simulink library "VIS_LIB_backup20190220"  (Simulink 8.6)
settings: Solver=ode45  StartTime=0.0  StopTime=10.0  RelTol=1e-3
undefined symbols (not defined in the file): AC, SIXOSEM_F_WD_AC_MASTER, VIS_LIB, WD2
libraries: cdsEpicsOut x104, cdsTP x55, cdsFilt x52, cdsFiltCtrl x23, cdsRms x23, cdsEpicsIn x16, STATE_BIO_MASTER x5, FOUROSEM_WD_AC_MASTER x4, cdsFunctionCall x2, TYPEB_MASTER x1, cdsEpicsBinIn x1, CRYP_TM_MASTER x1
(part 1 of 9)
settings Model: Creator=keiko  LastModifiedBy=controls

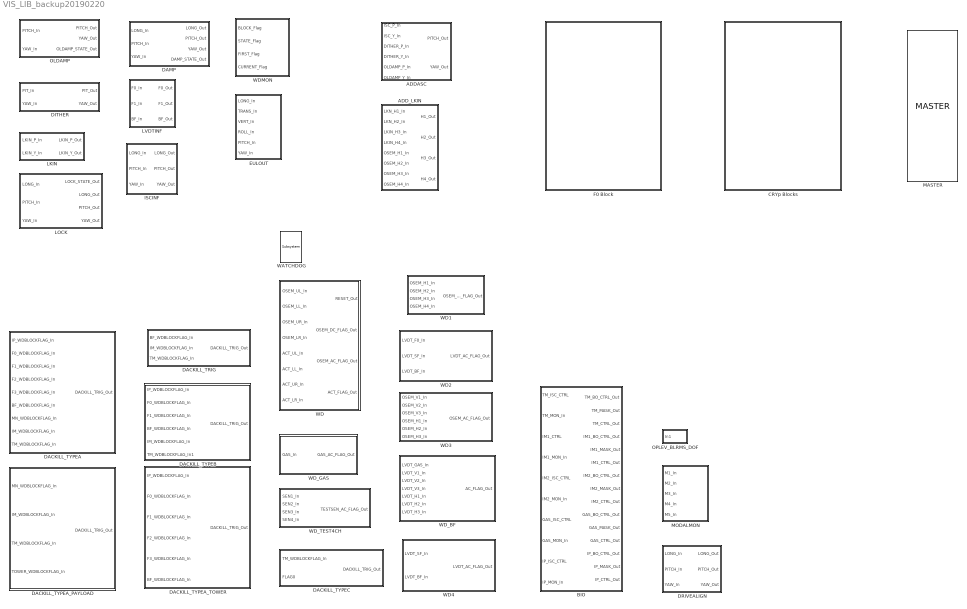
== system VIS_LIB_backup20190220 ==
  ADDASC : Subsystem
  ADD_LKIN : Subsystem
  BIO : Subsystem
  CRYp Blocks : Subsystem
  DACKILL_TRIG : Subsystem
  DACKILL_TYPEA : Subsystem
  DACKILL_TYPEA_PAYLOAD : Subsystem
  DACKILL_TYPEA_TOWER : Subsystem
  DACKILL_TYPEB : Subsystem
  "DACKILL_TYPEC " : Subsystem
  DAMP : Subsystem
  DITHER : Subsystem
  DRIVEALIGN : Subsystem
  EULOUT : Subsystem
  F0 Block : Subsystem
  ISCINF : Subsystem
  LKIN : Subsystem
  LOCK : Subsystem
  LVDTINF : Subsystem
  MASTER : CRYP_TM_MASTER/CRYP_TM_MASTER/MASTER
  MODALMON : Subsystem
  OLDAMP : Subsystem
  OPLEV_BLRMS_DOF : Subsystem
  WATCHDOG : cdsFunctionCall/Subsystem  Tag=cdsFunctionCall  Description=inline OSEMWATCHDOG $SUS_SRC/WATCHDOG.c
      settings: AttributesFormatString=%<Tag>\n%<Description>
  WD : Subsystem
  WD1 : Subsystem
  WD2 : Subsystem
  WD3 : Subsystem
  WD4 : Subsystem  AncestorBlock=VIS_LIB/WD2
  WDMON : Subsystem
  WD_BF : Subsystem
  WD_GAS : Subsystem
  WD_TEST4CH : Subsystem

== system VIS_LIB_backup20190220/ADDASC ==
  ISC_P_In : Inport
  ISC_Y_In : Inport  Port=2
  DITHER_P_In : Inport  Port=3
  DITHER_Y_In : Inport  Port=4
  OLDAMP_P_In : Inport  Port=5
  OLDAMP_Y_In : Inport  Port=6
  Sum3 : Sum  Inputs=+++
  Sum4 : Sum  Inputs=+++
  PITCH_Out : Outport
  YAW_Out : Outport  Port=2
  wires:
  OLDAMP_Y_In/1 -> Sum3/3
  DITHER_Y_In/1 -> Sum3/2
  DITHER_P_In/1 -> Sum4/2
  OLDAMP_P_In/1 -> Sum4/3
  Sum4/1 -> PITCH_Out/1
  ISC_Y_In/1 -> Sum3/1
  ISC_P_In/1 -> Sum4/1
  Sum3/1 -> YAW_Out/1

== system VIS_LIB_backup20190220/ADD_LKIN ==
  LKN_H1_In : Inport
  LKN_H2_In : Inport  Port=2
  LKIN_H3_In : Inport  Port=3
  LKIN_H4_In : Inport  Port=4
  OSEM_H1_In : Inport  Port=5
  OSEM_H2_In : Inport  Port=6
  OSEM_H3_In : Inport  Port=7
  OSEM_H4_In : Inport  Port=8
  Sum{,1,3..4} (4 alike) : Sum
  H1_Out : Outport
  H2_Out : Outport  Port=2
  H3_Out : Outport  Port=3
  H4_Out : Outport  Port=4
  wires:
  LKIN_H4_In/1 -> Sum1/1
  LKIN_H3_In/1 -> Sum3/1
  LKN_H2_In/1 -> Sum4/1
  Sum/1 -> H1_Out/1
  LKN_H1_In/1 -> Sum/1
  OSEM_H1_In/1 -> Sum/2
  Sum3/1 -> H3_Out/1
  Sum4/1 -> H2_Out/1
  OSEM_H3_In/1 -> Sum3/2
  OSEM_H2_In/1 -> Sum4/2
  Sum1/1 -> H4_Out/1
  OSEM_H4_In/1 -> Sum1/2

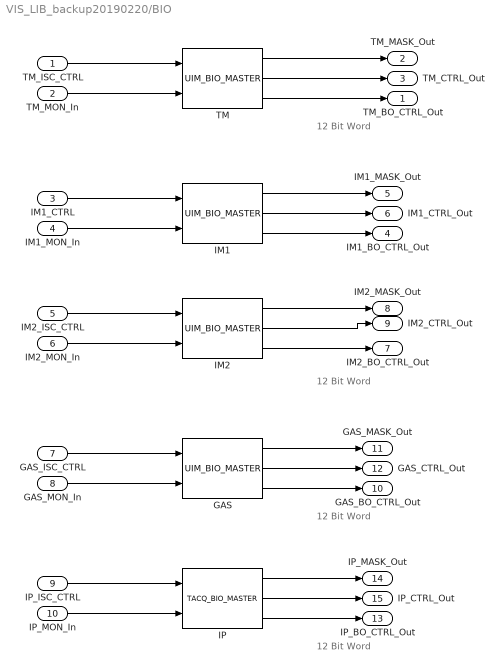
== system VIS_LIB_backup20190220/BIO ==
  note: 12 Bit Word
  note: 12 Bit Word
  note: 12 Bit Word
  note: 12 Bit Word
  TM_ISC_CTRL : Inport
  TM_MON_In : Inport  Port=2
  IM1_CTRL : Inport  Port=3
  IM1_MON_In : Inport  Port=4
  IM2_ISC_CTRL : Inport  Port=5
  IM2_MON_In : Inport  Port=6
  GAS_ISC_CTRL : Inport  Port=7
  GAS_MON_In : Inport  Port=8
  IP_ISC_CTRL : Inport  Port=9
  IP_MON_In : Inport  Port=10
  GAS : STATE_BIO_MASTER/UIM_BIO_MASTER
  IM1 : STATE_BIO_MASTER/UIM_BIO_MASTER
  IM2 : STATE_BIO_MASTER/UIM_BIO_MASTER
  IP : STATE_BIO_MASTER/TACQ_BIO_MASTER
  TM : STATE_BIO_MASTER/UIM_BIO_MASTER
  TM_BO_CTRL_Out : Outport
  TM_MASK_Out : Outport  Port=2
  TM_CTRL_Out : Outport  Port=3
  IM1_BO_CTRL_Out : Outport  Port=4
  IM1_MASK_Out : Outport  Port=5
  IM1_CTRL_Out : Outport  Port=6
  IM2_BO_CTRL_Out : Outport  Port=7
  IM2_MASK_Out : Outport  Port=8
  IM2_CTRL_Out : Outport  Port=9
  GAS_BO_CTRL_Out : Outport  Port=10
  GAS_MASK_Out : Outport  Port=11
  GAS_CTRL_Out : Outport  Port=12
  IP_BO_CTRL_Out : Outport  Port=13
  IP_MASK_Out : Outport  Port=14
  IP_CTRL_Out : Outport  Port=15
  wires:
  IP/3 -> IP_BO_CTRL_Out/1
  IP/2 -> IP_CTRL_Out/1
  IP/1 -> IP_MASK_Out/1
  GAS/3 -> GAS_BO_CTRL_Out/1
  GAS/2 -> GAS_CTRL_Out/1
  GAS/1 -> GAS_MASK_Out/1
  IM2/3 -> IM2_BO_CTRL_Out/1
  IM2/2 -> IM2_CTRL_Out/1
  IM2/1 -> IM2_MASK_Out/1
  IM1/3 -> IM1_BO_CTRL_Out/1
  IM1/2 -> IM1_CTRL_Out/1
  IM1/1 -> IM1_MASK_Out/1
  TM/3 -> TM_BO_CTRL_Out/1
  TM/2 -> TM_CTRL_Out/1
  TM/1 -> TM_MASK_Out/1
  IP_ISC_CTRL/1 -> IP/1
  IP_MON_In/1 -> IP/2
  GAS_ISC_CTRL/1 -> GAS/1
  GAS_MON_In/1 -> GAS/2
  IM2_ISC_CTRL/1 -> IM2/1
  IM2_MON_In/1 -> IM2/2
  IM1_MON_In/1 -> IM1/2
  IM1_CTRL/1 -> IM1/1
  TM_ISC_CTRL/1 -> TM/1
  TM_MON_In/1 -> TM/2

== system VIS_LIB_backup20190220/CRYp Blocks ==
  COILOUTF : Subsystem
  MASTER : Subsystem
  PSWD : Subsystem

== system VIS_LIB_backup20190220/DACKILL_TRIG ==
  note: WDBLOCKFLAG is zero (0) if OK,
      | non-zero if BAD
  note: AND is zero  (0) if all stages are OK
      | non-zero if BAD
  BF_WDBLOCKFLAG_In : Inport
  IM_WDBLOCKFLAG_In : Inport  Port=2
  TM_WDBLOCKFLAG_In : Inport  Port=3
  LogicalOperator1 : Logic  Operator=OR  Inputs=3  AllPortsSameDT=off  OutDataTypeStr=boolean
  STATE : cdsEpicsOut/Subsystem  Tag=cdsEpicsOutput  Description=|
      | Purpose:                                          
      | Output a FE signal to an EPICS channel.           
      |                                                   
      | Operation:                                        
      | Takes input value and passes it to EPICS record.  
      |                                                   
      | Usage:                                            
      | Name the part with the desired EPICS rrecord name.
      settings: AttributesFormatString=%<Tag>
  DACKILL_TRIG_Out : Outport
  wires:
  STATE/1 -> DACKILL_TRIG_Out/1
  BF_WDBLOCKFLAG_In/1 -> LogicalOperator1/1
  IM_WDBLOCKFLAG_In/1 -> LogicalOperator1/2
  TM_WDBLOCKFLAG_In/1 -> LogicalOperator1/3
  LogicalOperator1/1 -> STATE/1

== system VIS_LIB_backup20190220/DACKILL_TYPEA ==
  note: WDBLOCKFLAG is zero (0) if OK,
      | non-zero if BAD
  note: AND is zero  (0) if all stages are OK
      | non-zero if BAD
  IP_WDBLOCKFLAG_In : Inport
  F0_WDBLOCKFLAG_In : Inport  Port=2
  F1_WDBLOCKFLAG_In : Inport  Port=3
  F2_WDBLOCKFLAG_In : Inport  Port=4
  F3_WDBLOCKFLAG_In : Inport  Port=5
  BF_WDBLOCKFLAG_In : Inport  Port=6
  MN_WDBLOCKFLAG_In : Inport  Port=7
  IM_WDBLOCKFLAG_In : Inport  Port=8
  TM_WDBLOCKFLAG_In : Inport  Port=9
  LogicalOperator1 : Logic  Operator=OR  Inputs=9  AllPortsSameDT=off  OutDataTypeStr=boolean
  STATE : cdsEpicsOut/Subsystem  Tag=cdsEpicsOutput  Description=|
      | Purpose:                                          
      | Output a FE signal to an EPICS channel.           
      |                                                   
      | Operation:                                        
      | Takes input value and passes it to EPICS record.  
      |                                                   
      | Usage:                                            
      | Name the part with the desired EPICS rrecord name.
      settings: AttributesFormatString=%<Tag>
  DACKILL_TRIG_Out : Outport
  wires:
  STATE/1 -> DACKILL_TRIG_Out/1
  IP_WDBLOCKFLAG_In/1 -> LogicalOperator1/1
  F0_WDBLOCKFLAG_In/1 -> LogicalOperator1/2
  F1_WDBLOCKFLAG_In/1 -> LogicalOperator1/3
  LogicalOperator1/1 -> STATE/1
  IM_WDBLOCKFLAG_In/1 -> LogicalOperator1/8
  BF_WDBLOCKFLAG_In/1 -> LogicalOperator1/6
  TM_WDBLOCKFLAG_In/1 -> LogicalOperator1/9
  MN_WDBLOCKFLAG_In/1 -> LogicalOperator1/7
  F3_WDBLOCKFLAG_In/1 -> LogicalOperator1/5
  F2_WDBLOCKFLAG_In/1 -> LogicalOperator1/4

== system VIS_LIB_backup20190220/DACKILL_TYPEA_PAYLOAD ==
  note: WDBLOCKFLAG is zero (0) if OK,
      | non-zero if BAD
  note: AND is zero  (0) if all stages are OK
      | non-zero if BAD
  MN_WDBLOCKFLAG_In : Inport
  IM_WDBLOCKFLAG_In : Inport  Port=2
  TM_WDBLOCKFLAG_In : Inport  Port=3
  TOWER_WDBLOCKFLAG_In : Inport  Port=4
  LogicalOperator1 : Logic  Operator=OR  Inputs=3  AllPortsSameDT=off  OutDataTypeStr=boolean
  LogicalOperator2 : Logic  Operator=OR  AllPortsSameDT=off  OutDataTypeStr=boolean
  PAYLOAD_STATE : cdsEpicsOut/Subsystem  Tag=cdsEpicsOutput  Description=|
      | Purpose:                                          
      | Output a FE signal to an EPICS channel.           
      |                                                   
      | Operation:                                        
      | Takes input value and passes it to EPICS record.  
      |                                                   
      | Usage:                                            
      | Name the part with the desired EPICS rrecord name.
      settings: AttributesFormatString=%<Tag>
  STATE : cdsEpicsOut/Subsystem  Tag=cdsEpicsOutput  Description=|
      | Purpose:                                          
      | Output a FE signal to an EPICS channel.           
      |                                                   
      | Operation:                                        
      | Takes input value and passes it to EPICS record.  
      |                                                   
      | Usage:                                            
      | Name the part with the desired EPICS rrecord name.
      settings: AttributesFormatString=%<Tag>
  DACKILL_TRIG_Out : Outport
  wires:
  LogicalOperator1/1 -> PAYLOAD_STATE/1
  IM_WDBLOCKFLAG_In/1 -> LogicalOperator1/2
  TM_WDBLOCKFLAG_In/1 -> LogicalOperator1/3
  MN_WDBLOCKFLAG_In/1 -> LogicalOperator1/1
  TOWER_WDBLOCKFLAG_In/1 -> LogicalOperator2/2
  PAYLOAD_STATE/1 -> LogicalOperator2/1
  LogicalOperator2/1 -> STATE/1
  STATE/1 -> DACKILL_TRIG_Out/1

== system VIS_LIB_backup20190220/DACKILL_TYPEA_TOWER ==
  note: WDBLOCKFLAG is zero (0) if OK,
      | non-zero if BAD
  note: AND is zero  (0) if all stages are OK
      | non-zero if BAD
  IP_WDBLOCKFLAG_In : Inport
  F0_WDBLOCKFLAG_In : Inport  Port=2
  F1_WDBLOCKFLAG_In : Inport  Port=3
  F2_WDBLOCKFLAG_In : Inport  Port=4
  F3_WDBLOCKFLAG_In : Inport  Port=5
  BF_WDBLOCKFLAG_In : Inport  Port=6
  LogicalOperator1 : Logic  Operator=OR  Inputs=6  AllPortsSameDT=off  OutDataTypeStr=boolean
  STATE : cdsEpicsOut/Subsystem  Tag=cdsEpicsOutput  Description=|
      | Purpose:                                          
      | Output a FE signal to an EPICS channel.           
      |                                                   
      | Operation:                                        
      | Takes input value and passes it to EPICS record.  
      |                                                   
      | Usage:                                            
      | Name the part with the desired EPICS rrecord name.
      settings: AttributesFormatString=%<Tag>
  DACKILL_TRIG_Out : Outport
  wires:
  STATE/1 -> DACKILL_TRIG_Out/1
  IP_WDBLOCKFLAG_In/1 -> LogicalOperator1/1
  F0_WDBLOCKFLAG_In/1 -> LogicalOperator1/2
  F1_WDBLOCKFLAG_In/1 -> LogicalOperator1/3
  LogicalOperator1/1 -> STATE/1
  BF_WDBLOCKFLAG_In/1 -> LogicalOperator1/6
  F3_WDBLOCKFLAG_In/1 -> LogicalOperator1/5
  F2_WDBLOCKFLAG_In/1 -> LogicalOperator1/4

== system VIS_LIB_backup20190220/DACKILL_TYPEB ==
  note: WDBLOCKFLAG is zero (0) if OK,
      | non-zero if BAD
  note: AND is zero  (0) if all stages are OK
      | non-zero if BAD
  IP_WDBLOCKFLAG_In : Inport
  F0_WDBLOCKFLAG_In : Inport  Port=2
  F1_WDBLOCKFLAG_In : Inport  Port=3
  BF_WDBLOCKFLAG_In : Inport  Port=4
  IM_WDBLOCKFLAG_In : Inport  Port=5
  TM_WDBLOCKFLAG_In1 : Inport  Port=6
  LogicalOperator1 : Logic  Operator=OR  Inputs=6  AllPortsSameDT=off  OutDataTypeStr=boolean
  STATE : cdsEpicsOut/Subsystem  Tag=cdsEpicsOutput  Description=|
      | Purpose:                                          
      | Output a FE signal to an EPICS channel.           
      |                                                   
      | Operation:                                        
      | Takes input value and passes it to EPICS record.  
      |                                                   
      | Usage:                                            
      | Name the part with the desired EPICS rrecord name.
      settings: AttributesFormatString=%<Tag>
  DACKILL_TRIG_Out : Outport
  wires:
  STATE/1 -> DACKILL_TRIG_Out/1
  IP_WDBLOCKFLAG_In/1 -> LogicalOperator1/1
  F0_WDBLOCKFLAG_In/1 -> LogicalOperator1/2
  F1_WDBLOCKFLAG_In/1 -> LogicalOperator1/3
  LogicalOperator1/1 -> STATE/1
  IM_WDBLOCKFLAG_In/1 -> LogicalOperator1/5
  BF_WDBLOCKFLAG_In/1 -> LogicalOperator1/4
  TM_WDBLOCKFLAG_In1/1 -> LogicalOperator1/6

== system VIS_LIB_backup20190220/DACKILL_TYPEC  ==
  note: WDBLOCKFLAG is zero (0) if OK,
      | non-zero if BAD
  note: AND is zero  (0) if all stages are OK
      | non-zero if BAD
  TM_WDBLOCKFLAG_In : Inport
  FLAG0 : Inport  Port=2
  LogicalOperator1 : Logic  Operator=OR  AllPortsSameDT=off  OutDataTypeStr=boolean
  STATE : cdsEpicsOut/Subsystem  Tag=cdsEpicsOutput  Description=|
      | Purpose:                                          
      | Output a FE signal to an EPICS channel.           
      |                                                   
      | Operation:                                        
      | Takes input value and passes it to EPICS record.  
      |                                                   
      | Usage:                                            
      | Name the part with the desired EPICS rrecord name.
      settings: AttributesFormatString=%<Tag>
  DACKILL_TRIG_Out : Outport
  wires:
  STATE/1 -> DACKILL_TRIG_Out/1
  TM_WDBLOCKFLAG_In/1 -> LogicalOperator1/2
  LogicalOperator1/1 -> STATE/1
  FLAG0/1 -> LogicalOperator1/1

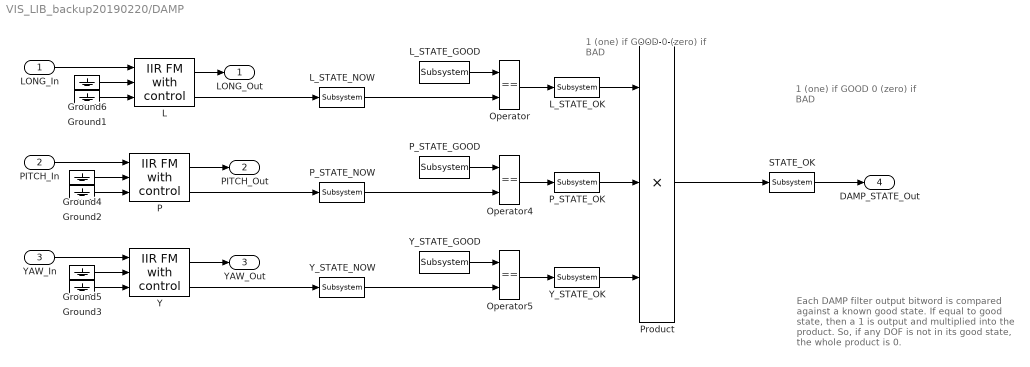
== system VIS_LIB_backup20190220/DAMP ==
  note: 1 (one) if GOOD
      | 0 (zero) if BAD
  note: 1 (one) if GOOD
      | 0 (zero) if BAD
  note: Each DAMP filter output bitword is
      | compared against a known good state.
      | If equal to good state, then a 1 is output
      | and multiplied into the product. So, if any DOF
      | is not in its good state, the whole product is 0.
  LONG_In : Inport
  PITCH_In : Inport  Port=2
  YAW_In : Inport  Port=3
  Ground{1..6} (6 alike) : Ground
  L : cdsFiltCtrl/IIR FM with control  Tag=cdsFiltCtrl  Description=|
      | cdsFiltCntrl is the standard IIR filter module (exactly the same as cdsFilt) but with added control data output 'Ctrl'. Filter module digital signal output appears on the first output, which is called 'Val'. 'Ctrl' output has a bit pattern encoding the state of filter's on/off switches (FM1 through FM10). The bit values are:
      |                                                                                                                                                                                                                                                                                                                                       
      | module 	hex	dec                                                                                                                                                                                                                                                                                                                       
      | -----------------------                                                                                                                                                                                                                                                                                                               
      | FM1	0x20                    32                                                                                                                                                                                                                                                                                                        
      | FM2	0x80                     128                                                                                                                                                                                                                                                                                                      
      | FM3	0x200                   512                                                                                                                                                                                                                                                                                                       
      | FM4	0x800                   2048                                                                                                                                                                                                                                                                                                      
      | FM5	0x2000                 8192                                                                                                                                                                                                                                                                                                       
      | FM6	0x8000                 32768                                                                                                                                                                                                                                                                                                      
      | FM7	0x20000                131072                                                                                                                                                                                                                                                                                                     
      | FM8	0x80000                 524288                                                                                                                                                                                                                                                                                                    
      | FM9	0x200000               2097152                                                                                                                                                                                                                                                                                                    
      | FM10	0x800000               8388608                                                                                                                                                                                                                                                                                                   
      |                                                                                                                                                                                                                                                                                                                                       
      | This bit data can be used to drive some other switches or it can be output using a binary I/O module.
      settings: AttributesFormatString=%<Tag>
  L_STATE_GOOD : cdsEpicsIn/Subsystem  Tag=cdsEpicsIn  Description=|
      | Purpose:                                                                              
      | Create an EPICS input channel connection to the FE realtime controls.                 
      |                                                                                       
      | Operation:                                                                            
      | Outputs value from an EPICS ai record. Value is floating point with a precision of 3..
      |                                                                                       
      | Usage:                                                                                
      | Name the part with the desired EPICS channel name.
      settings: AttributesFormatString=%<Tag>
  L_STATE_NOW : cdsEpicsOut/Subsystem  Tag=cdsEpicsOutput  Description=|
      | Purpose:                                          
      | Output a FE signal to an EPICS channel.           
      |                                                   
      | Operation:                                        
      | Takes input value and passes it to EPICS record.  
      |                                                   
      | Usage:                                            
      | Name the part with the desired EPICS rrecord name.
      settings: AttributesFormatString=%<Tag>
  L_STATE_OK : cdsEpicsOut/Subsystem  Tag=cdsEpicsOutput  Description=|
      | Purpose:                                          
      | Output a FE signal to an EPICS channel.           
      |                                                   
      | Operation:                                        
      | Takes input value and passes it to EPICS record.  
      |                                                   
      | Usage:                                            
      | Name the part with the desired EPICS rrecord name.
      settings: AttributesFormatString=%<Tag>
  Operator : RelationalOperator  Operator===  OutDataTypeStr=boolean
  Operator4 : RelationalOperator  Operator===  OutDataTypeStr=boolean
  Operator5 : RelationalOperator  Operator===  OutDataTypeStr=boolean
  P : cdsFiltCtrl/IIR FM with control  Tag=cdsFiltCtrl  Description=|
      | cdsFiltCntrl is the standard IIR filter module (exactly the same as cdsFilt) but with added control data output 'Ctrl'. Filter module digital signal output appears on the first output, which is called 'Val'. 'Ctrl' output has a bit pattern encoding the state of filter's on/off switches (FM1 through FM10). The bit values are:
      |                                                                                                                                                                                                                                                                                                                                       
      | module 	hex	dec                                                                                                                                                                                                                                                                                                                       
      | -----------------------                                                                                                                                                                                                                                                                                                               
      | FM1	0x20                    32                                                                                                                                                                                                                                                                                                        
      | FM2	0x80                     128                                                                                                                                                                                                                                                                                                      
      | FM3	0x200                   512                                                                                                                                                                                                                                                                                                       
      | FM4	0x800                   2048                                                                                                                                                                                                                                                                                                      
      | FM5	0x2000                 8192                                                                                                                                                                                                                                                                                                       
      | FM6	0x8000                 32768                                                                                                                                                                                                                                                                                                      
      | FM7	0x20000                131072                                                                                                                                                                                                                                                                                                     
      | FM8	0x80000                 524288                                                                                                                                                                                                                                                                                                    
      | FM9	0x200000               2097152                                                                                                                                                                                                                                                                                                    
      | FM10	0x800000               8388608                                                                                                                                                                                                                                                                                                   
      |                                                                                                                                                                                                                                                                                                                                       
      | This bit data can be used to drive some other switches or it can be output using a binary I/O module.
      settings: AttributesFormatString=%<Tag>
  P_STATE_GOOD : cdsEpicsIn/Subsystem  Tag=cdsEpicsIn  Description=|
      | Purpose:                                                                              
      | Create an EPICS input channel connection to the FE realtime controls.                 
      |                                                                                       
      | Operation:                                                                            
      | Outputs value from an EPICS ai record. Value is floating point with a precision of 3..
      |                                                                                       
      | Usage:                                                                                
      | Name the part with the desired EPICS channel name.
      settings: AttributesFormatString=%<Tag>
  P_STATE_NOW : cdsEpicsOut/Subsystem  Tag=cdsEpicsOutput  Description=|
      | Purpose:                                          
      | Output a FE signal to an EPICS channel.           
      |                                                   
      | Operation:                                        
      | Takes input value and passes it to EPICS record.  
      |                                                   
      | Usage:                                            
      | Name the part with the desired EPICS rrecord name.
      settings: AttributesFormatString=%<Tag>
  P_STATE_OK : cdsEpicsOut/Subsystem  Tag=cdsEpicsOutput  Description=|
      | Purpose:                                          
      | Output a FE signal to an EPICS channel.           
      |                                                   
      | Operation:                                        
      | Takes input value and passes it to EPICS record.  
      |                                                   
      | Usage:                                            
      | Name the part with the desired EPICS rrecord name.
      settings: AttributesFormatString=%<Tag>
  Product : Product  Inputs=3  RndMeth=Zero
  STATE_OK : cdsEpicsOut/Subsystem  Tag=cdsEpicsOutput  Description=|
      | Purpose:                                          
      | Output a FE signal to an EPICS channel.           
      |                                                   
      | Operation:                                        
      | Takes input value and passes it to EPICS record.  
      |                                                   
      | Usage:                                            
      | Name the part with the desired EPICS rrecord name.
      settings: AttributesFormatString=%<Tag>
  Y : cdsFiltCtrl/IIR FM with control  Tag=cdsFiltCtrl  Description=|
      | cdsFiltCntrl is the standard IIR filter module (exactly the same as cdsFilt) but with added control data output 'Ctrl'. Filter module digital signal output appears on the first output, which is called 'Val'. 'Ctrl' output has a bit pattern encoding the state of filter's on/off switches (FM1 through FM10). The bit values are:
      |                                                                                                                                                                                                                                                                                                                                       
      | module 	hex	dec                                                                                                                                                                                                                                                                                                                       
      | -----------------------                                                                                                                                                                                                                                                                                                               
      | FM1	0x20                    32                                                                                                                                                                                                                                                                                                        
      | FM2	0x80                     128                                                                                                                                                                                                                                                                                                      
      | FM3	0x200                   512                                                                                                                                                                                                                                                                                                       
      | FM4	0x800                   2048                                                                                                                                                                                                                                                                                                      
      | FM5	0x2000                 8192                                                                                                                                                                                                                                                                                                       
      | FM6	0x8000                 32768                                                                                                                                                                                                                                                                                                      
      | FM7	0x20000                131072                                                                                                                                                                                                                                                                                                     
      | FM8	0x80000                 524288                                                                                                                                                                                                                                                                                                    
      | FM9	0x200000               2097152                                                                                                                                                                                                                                                                                                    
      | FM10	0x800000               8388608                                                                                                                                                                                                                                                                                                   
      |                                                                                                                                                                                                                                                                                                                                       
      | This bit data can be used to drive some other switches or it can be output using a binary I/O module.
      settings: AttributesFormatString=%<Tag>
  Y_STATE_GOOD : cdsEpicsIn/Subsystem  Tag=cdsEpicsIn  Description=|
      | Purpose:                                                                              
      | Create an EPICS input channel connection to the FE realtime controls.                 
      |                                                                                       
      | Operation:                                                                            
      | Outputs value from an EPICS ai record. Value is floating point with a precision of 3..
      |                                                                                       
      | Usage:                                                                                
      | Name the part with the desired EPICS channel name.
      settings: AttributesFormatString=%<Tag>
  Y_STATE_NOW : cdsEpicsOut/Subsystem  Tag=cdsEpicsOutput  Description=|
      | Purpose:                                          
      | Output a FE signal to an EPICS channel.           
      |                                                   
      | Operation:                                        
      | Takes input value and passes it to EPICS record.  
      |                                                   
      | Usage:                                            
      | Name the part with the desired EPICS rrecord name.
      settings: AttributesFormatString=%<Tag>
  Y_STATE_OK : cdsEpicsOut/Subsystem  Tag=cdsEpicsOutput  Description=|
      | Purpose:                                          
      | Output a FE signal to an EPICS channel.           
      |                                                   
      | Operation:                                        
      | Takes input value and passes it to EPICS record.  
      |                                                   
      | Usage:                                            
      | Name the part with the desired EPICS rrecord name.
      settings: AttributesFormatString=%<Tag>
  LONG_Out : Outport
  PITCH_Out : Outport  Port=2
  YAW_Out : Outport  Port=3
  DAMP_STATE_Out : Outport  Port=4
  wires:
  STATE_OK/1 -> DAMP_STATE_Out/1
  Y_STATE_NOW/1 -> Operator5/2
  P_STATE_NOW/1 -> Operator4/2
  L_STATE_NOW/1 -> Operator/2
  Y_STATE_OK/1 -> Product/3
  P_STATE_OK/1 -> Product/2
  L_STATE_OK/1 -> Product/1
  Operator5/1 -> Y_STATE_OK/1
  Operator4/1 -> P_STATE_OK/1
  Operator/1 -> L_STATE_OK/1
  Product/1 -> STATE_OK/1
  Y/2 -> Y_STATE_NOW/1
  Y_STATE_GOOD/1 -> Operator5/1
  P/2 -> P_STATE_NOW/1
  P_STATE_GOOD/1 -> Operator4/1
  L/2 -> L_STATE_NOW/1
  L_STATE_GOOD/1 -> Operator/1
  PITCH_In/1 -> P/1
  YAW_In/1 -> Y/1
  L/1 -> LONG_Out/1
  LONG_In/1 -> L/1
  Ground5/1 -> Y/2
  Ground4/1 -> P/2
  Ground6/1 -> L/2
  Y/1 -> YAW_Out/1
  P/1 -> PITCH_Out/1
  Ground1/1 -> L/3
  Ground2/1 -> P/3
  Ground3/1 -> Y/3

== system VIS_LIB_backup20190220/DITHER ==
  PIT_In : Inport
  YAW_In : Inport  Port=2
  P : cdsFilt/Subsystem  Tag=cdsFilt  Description=|
      | Purpose:                                                                                                                                                                                                                                  
      | Standard CDS IIR filter module.                                                                                                                                                                                                           
      |                                                                                                                                                                                                                                           
      | Operation:                                                                                                                                                                                                                                
      | Consists of 10 second order section IIR filters, plus a ramped gain stage. In FE code, also provides pre-defined test points and excitation channel inputs. The filter coefficients are defined in the LIGO system using the 'foton' tool.
      |                                                                                                                                                                                                                                           
      | Usage:                                                                                                                                                                                                                                    
      | Name the part with the desired filter module name.
      settings: AttributesFormatString=%<Tag>
  Y : cdsFilt/Subsystem  Tag=cdsFilt  Description=|
      | Purpose:                                                                                                                                                                                                                                  
      | Standard CDS IIR filter module.                                                                                                                                                                                                           
      |                                                                                                                                                                                                                                           
      | Operation:                                                                                                                                                                                                                                
      | Consists of 10 second order section IIR filters, plus a ramped gain stage. In FE code, also provides pre-defined test points and excitation channel inputs. The filter coefficients are defined in the LIGO system using the 'foton' tool.
      |                                                                                                                                                                                                                                           
      | Usage:                                                                                                                                                                                                                                    
      | Name the part with the desired filter module name.
      settings: AttributesFormatString=%<Tag>
  PIT_Out : Outport
  YAW_Out : Outport  Port=2
  wires:
  P/1 -> PIT_Out/1
  YAW_In/1 -> Y/1
  Y/1 -> YAW_Out/1
  PIT_In/1 -> P/1
